simulink model "model_cnn"  (R2020a)
settings: Solver=VariableStepAuto  StartTime=0.0  StopTime=1e6/fs  RelTol=1e-3
PreLoadFcn:
  | setup_imports;
  | %dense2_numerictype = fixdt(1,18,10);
  | %conv1_numerictype = fixdt(1,18,21);
InitFcn:
  | % Intermediate signal dimensions
  | input_dim = [1, 2, 128];
  | layer1_dim = hInterConvLayerDims([1,3,1,64],input_dim,1); % dims : [C,H,W]
  | layer2_dim = hInterConvLayerDims([2,3,64,16],layer1_dim,1);% dims : [C,H,W]
  | layer3_dim = [1,128];
  | 
  | % Conv Layer 1 dimensions
  | conv1_dims = struct(...
  |     'input_dim',    input_dim,...       input_dim = C,H,W
  |     'filter_dim',   [1, 3, 1, 64],...  filter_dim = K,J,C,N
  |     'stride',       1,...
  |     'row_output',   3,...
  |     'output_dim',   layer1_dim);
  | 
  | % Conv Layer 2 dimensions
  | conv2_dims = struct(...
  |     'input_dim',    layer1_dim,...      input = C,H.W
  |     'filter_dim',   [2, 3, 64, 16],...  filter_dim = K,J,C,N
  |     'stride',       1,...
  |     'row_output',   2*3*64,...
  |     'output_dim',   layer2_dim);
  | 
  | % Dense Layer 1 dimensions
  | dense1_dims = struct(...
  |     'input_dim',    layer2_dim,...      input = C,H,W
  |     'weight_dim',   [1984, 128],...     weight_dim = H,W
  |     'output_dim',   layer3_dim);
  | 
  | % Load saved weights and input
  | setup_imports;
  | 
  | fs = 128e6;
  | fs_axi = 100e6;
  | R = 32;
values from neighbouring files (symbols this model uses):
  datatypeInput = X_test.numerictype    [setup_imports.m]
  gemm_wconv1 = fi(hInterleaveFilters(Wconv1),1,16)    [setup_imports.m]
  gemm_wconv2 = fi(hInterleaveFilters(Wconv2),1,16)    [setup_imports.m]
  wdense1 = fi(Wdense1,1,16)    [setup_imports.m]
  wdense2 = fi(Wdense2,1,16)    [setup_imports.m]
undefined symbols (not defined in the file or in its folder): ltehdlRAMinitPO2
libraries: hdlsllib x1022, dspsigops x3, dspsrcs4 x2
(part 22 of 23)

== system model_cnn/HDL CNN Model/Conv Layer 2/Filter Matrix Multiplier1/ParallelMACs 9/MAC10 ==
  countWeights : Inport
  samplesIn : Inport  Port=2
  validIn : Inport  Port=3
  Data Type Conversion : DataTypeConversion  OutDataTypeStr=datatypeLayer2
  Multiply-Accumulate : hdlsllib/HDL Operations/Multiply-Accumulate  opMode=Streaming - using Number of Samples  initValueSetting=Dialog  initValue=0  initValueSetting2=Dialog  initValue2=0  initValueSetting3=Dialog  initValue3=0  num_samples=24  RndMeth2=Floor  RndMeth3=Floor  OutDataTypeStr=gemm_wconv2.numerictype  datatype2=Inherit: Inherit via back propagation  datatype3=accumoutdatatype2  validOut=on  endInandOut=on  startOut=on  countOut=on  dim=-1  DoSatur=off  parallel=off
      settings: SourceProductBaseCode=SL
  Terminator : Terminator
  Terminator1 : Terminator
  Terminator2 : Terminator
  dataOut : Outport
  wires:
  countWeights/1 -> Multiply-Accumulate/2
  ? -> Terminator2/1
  samplesIn/1 -> Multiply-Accumulate/1
  Multiply-Accumulate/1 -> Data Type Conversion/1
  ? -> Terminator/1
  ? -> Terminator1/1
  validIn/1 -> ?
  Data Type Conversion/1 -> dataOut/1

== system model_cnn/HDL CNN Model/Conv Layer 2/Filter Matrix Multiplier1/ParallelMACs 9/MAC11 ==
  countWeights : Inport
  samplesIn : Inport  Port=2
  validIn : Inport  Port=3
  Data Type Conversion : DataTypeConversion  OutDataTypeStr=datatypeLayer2
  Multiply-Accumulate : hdlsllib/HDL Operations/Multiply-Accumulate  opMode=Streaming - using Number of Samples  initValueSetting=Dialog  initValue=0  initValueSetting2=Dialog  initValue2=0  initValueSetting3=Dialog  initValue3=0  num_samples=24  RndMeth2=Floor  RndMeth3=Floor  OutDataTypeStr=gemm_wconv2.numerictype  datatype2=Inherit: Inherit via back propagation  datatype3=accumoutdatatype2  validOut=on  endInandOut=on  startOut=on  countOut=on  dim=-1  DoSatur=off  parallel=off
      settings: SourceProductBaseCode=SL
  Terminator : Terminator
  Terminator1 : Terminator
  Terminator2 : Terminator
  dataOut : Outport
  wires:
  countWeights/1 -> Multiply-Accumulate/2
  ? -> Terminator2/1
  samplesIn/1 -> Multiply-Accumulate/1
  Multiply-Accumulate/1 -> Data Type Conversion/1
  ? -> Terminator/1
  ? -> Terminator1/1
  validIn/1 -> ?
  Data Type Conversion/1 -> dataOut/1

== system model_cnn/HDL CNN Model/Conv Layer 2/Filter Matrix Multiplier1/ParallelMACs 9/MAC12 ==
  countWeights : Inport
  samplesIn : Inport  Port=2
  validIn : Inport  Port=3
  Data Type Conversion : DataTypeConversion  OutDataTypeStr=datatypeLayer2
  Multiply-Accumulate : hdlsllib/HDL Operations/Multiply-Accumulate  opMode=Streaming - using Number of Samples  initValueSetting=Dialog  initValue=0  initValueSetting2=Dialog  initValue2=0  initValueSetting3=Dialog  initValue3=0  num_samples=24  RndMeth2=Floor  RndMeth3=Floor  OutDataTypeStr=gemm_wconv2.numerictype  datatype2=Inherit: Inherit via back propagation  datatype3=accumoutdatatype2  validOut=on  endInandOut=on  startOut=on  countOut=on  dim=-1  DoSatur=off  parallel=off
      settings: SourceProductBaseCode=SL
  Terminator : Terminator
  Terminator1 : Terminator
  Terminator2 : Terminator
  dataOut : Outport
  wires:
  countWeights/1 -> Multiply-Accumulate/2
  ? -> Terminator2/1
  samplesIn/1 -> Multiply-Accumulate/1
  Multiply-Accumulate/1 -> Data Type Conversion/1
  ? -> Terminator/1
  ? -> Terminator1/1
  validIn/1 -> ?
  Data Type Conversion/1 -> dataOut/1

== system model_cnn/HDL CNN Model/Conv Layer 2/Filter Matrix Multiplier1/ParallelMACs 9/MAC13 ==
  countWeights : Inport
  samplesIn : Inport  Port=2
  validIn : Inport  Port=3
  Data Type Conversion : DataTypeConversion  OutDataTypeStr=datatypeLayer2
  Multiply-Accumulate : hdlsllib/HDL Operations/Multiply-Accumulate  opMode=Streaming - using Number of Samples  initValueSetting=Dialog  initValue=0  initValueSetting2=Dialog  initValue2=0  initValueSetting3=Dialog  initValue3=0  num_samples=24  RndMeth2=Floor  RndMeth3=Floor  OutDataTypeStr=gemm_wconv2.numerictype  datatype2=Inherit: Inherit via back propagation  datatype3=accumoutdatatype2  validOut=on  endInandOut=on  startOut=on  countOut=on  dim=-1  DoSatur=off  parallel=off
      settings: SourceProductBaseCode=SL
  Terminator : Terminator
  Terminator1 : Terminator
  Terminator2 : Terminator
  dataOut : Outport
  wires:
  countWeights/1 -> Multiply-Accumulate/2
  ? -> Terminator2/1
  samplesIn/1 -> Multiply-Accumulate/1
  Multiply-Accumulate/1 -> Data Type Conversion/1
  ? -> Terminator/1
  ? -> Terminator1/1
  validIn/1 -> ?
  Data Type Conversion/1 -> dataOut/1

== system model_cnn/HDL CNN Model/Conv Layer 2/Filter Matrix Multiplier1/ParallelMACs 9/MAC14 ==
  countWeights : Inport
  samplesIn : Inport  Port=2
  validIn : Inport  Port=3
  Data Type Conversion : DataTypeConversion  OutDataTypeStr=datatypeLayer2
  Multiply-Accumulate : hdlsllib/HDL Operations/Multiply-Accumulate  opMode=Streaming - using Number of Samples  initValueSetting=Dialog  initValue=0  initValueSetting2=Dialog  initValue2=0  initValueSetting3=Dialog  initValue3=0  num_samples=24  RndMeth2=Floor  RndMeth3=Floor  OutDataTypeStr=gemm_wconv2.numerictype  datatype2=Inherit: Inherit via back propagation  datatype3=accumoutdatatype2  validOut=on  endInandOut=on  startOut=on  countOut=on  dim=-1  DoSatur=off  parallel=off
      settings: SourceProductBaseCode=SL
  Terminator : Terminator
  Terminator1 : Terminator
  Terminator2 : Terminator
  dataOut : Outport
  wires:
  countWeights/1 -> Multiply-Accumulate/2
  ? -> Terminator2/1
  samplesIn/1 -> Multiply-Accumulate/1
  Multiply-Accumulate/1 -> Data Type Conversion/1
  ? -> Terminator/1
  ? -> Terminator1/1
  validIn/1 -> ?
  Data Type Conversion/1 -> dataOut/1

== system model_cnn/HDL CNN Model/Conv Layer 2/Filter Matrix Multiplier1/ParallelMACs 9/MAC15 ==
  countWeights : Inport
  samplesIn : Inport  Port=2
  validIn : Inport  Port=3
  Data Type Conversion : DataTypeConversion  OutDataTypeStr=datatypeLayer2
  Multiply-Accumulate : hdlsllib/HDL Operations/Multiply-Accumulate  opMode=Streaming - using Number of Samples  initValueSetting=Dialog  initValue=0  initValueSetting2=Dialog  initValue2=0  initValueSetting3=Dialog  initValue3=0  num_samples=24  RndMeth2=Floor  RndMeth3=Floor  OutDataTypeStr=gemm_wconv2.numerictype  datatype2=Inherit: Inherit via back propagation  datatype3=accumoutdatatype2  validOut=on  endInandOut=on  startOut=on  countOut=on  dim=-1  DoSatur=off  parallel=off
      settings: SourceProductBaseCode=SL
  Terminator : Terminator
  Terminator1 : Terminator
  Terminator2 : Terminator
  dataOut : Outport
  wires:
  countWeights/1 -> Multiply-Accumulate/2
  ? -> Terminator2/1
  samplesIn/1 -> Multiply-Accumulate/1
  Multiply-Accumulate/1 -> Data Type Conversion/1
  ? -> Terminator/1
  ? -> Terminator1/1
  validIn/1 -> ?
  Data Type Conversion/1 -> dataOut/1

== system model_cnn/HDL CNN Model/Conv Layer 2/Filter Matrix Multiplier1/ParallelMACs 9/MAC2 ==
  countWeights : Inport
  samplesIn : Inport  Port=2
  validIn : Inport  Port=3
  Data Type Conversion : DataTypeConversion  OutDataTypeStr=datatypeLayer2
  Multiply-Accumulate : hdlsllib/HDL Operations/Multiply-Accumulate  opMode=Streaming - using Number of Samples  initValueSetting=Dialog  initValue=0  initValueSetting2=Dialog  initValue2=0  initValueSetting3=Dialog  initValue3=0  num_samples=24  RndMeth2=Floor  RndMeth3=Floor  OutDataTypeStr=gemm_wconv2.numerictype  datatype2=Inherit: Inherit via back propagation  datatype3=accumoutdatatype2  validOut=on  endInandOut=on  startOut=on  countOut=on  dim=-1  DoSatur=off  parallel=off
      settings: SourceProductBaseCode=SL
  Terminator : Terminator
  Terminator1 : Terminator
  Terminator2 : Terminator
  dataOut : Outport
  wires:
  countWeights/1 -> Multiply-Accumulate/2
  ? -> Terminator2/1
  samplesIn/1 -> Multiply-Accumulate/1
  Multiply-Accumulate/1 -> Data Type Conversion/1
  ? -> Terminator/1
  ? -> Terminator1/1
  validIn/1 -> ?
  Data Type Conversion/1 -> dataOut/1

== system model_cnn/HDL CNN Model/Conv Layer 2/Filter Matrix Multiplier1/ParallelMACs 9/MAC3 ==
  countWeights : Inport
  samplesIn : Inport  Port=2
  validIn : Inport  Port=3
  Data Type Conversion : DataTypeConversion  OutDataTypeStr=datatypeLayer2
  Multiply-Accumulate : hdlsllib/HDL Operations/Multiply-Accumulate  opMode=Streaming - using Number of Samples  initValueSetting=Dialog  initValue=0  initValueSetting2=Dialog  initValue2=0  initValueSetting3=Dialog  initValue3=0  num_samples=24  RndMeth2=Floor  RndMeth3=Floor  OutDataTypeStr=gemm_wconv2.numerictype  datatype2=Inherit: Inherit via back propagation  datatype3=accumoutdatatype2  validOut=on  endInandOut=on  startOut=on  countOut=on  dim=-1  DoSatur=off  parallel=off
      settings: SourceProductBaseCode=SL
  Terminator : Terminator
  Terminator1 : Terminator
  Terminator2 : Terminator
  dataOut : Outport
  wires:
  countWeights/1 -> Multiply-Accumulate/2
  ? -> Terminator2/1
  samplesIn/1 -> Multiply-Accumulate/1
  Multiply-Accumulate/1 -> Data Type Conversion/1
  ? -> Terminator/1
  ? -> Terminator1/1
  validIn/1 -> ?
  Data Type Conversion/1 -> dataOut/1

== system model_cnn/HDL CNN Model/Conv Layer 2/Filter Matrix Multiplier1/ParallelMACs 9/MAC4 ==
  countWeights : Inport
  samplesIn : Inport  Port=2
  validIn : Inport  Port=3
  Data Type Conversion : DataTypeConversion  OutDataTypeStr=datatypeLayer2
  Multiply-Accumulate : hdlsllib/HDL Operations/Multiply-Accumulate  opMode=Streaming - using Number of Samples  initValueSetting=Dialog  initValue=0  initValueSetting2=Dialog  initValue2=0  initValueSetting3=Dialog  initValue3=0  num_samples=24  RndMeth2=Floor  RndMeth3=Floor  OutDataTypeStr=gemm_wconv2.numerictype  datatype2=Inherit: Inherit via back propagation  datatype3=accumoutdatatype2  validOut=on  endInandOut=on  startOut=on  countOut=on  dim=-1  DoSatur=off  parallel=off
      settings: SourceProductBaseCode=SL
  Terminator : Terminator
  Terminator1 : Terminator
  Terminator2 : Terminator
  dataOut : Outport
  wires:
  countWeights/1 -> Multiply-Accumulate/2
  ? -> Terminator2/1
  samplesIn/1 -> Multiply-Accumulate/1
  Multiply-Accumulate/1 -> Data Type Conversion/1
  ? -> Terminator/1
  ? -> Terminator1/1
  validIn/1 -> ?
  Data Type Conversion/1 -> dataOut/1

== system model_cnn/HDL CNN Model/Conv Layer 2/Filter Matrix Multiplier1/ParallelMACs 9/MAC5 ==
  countWeights : Inport
  samplesIn : Inport  Port=2
  validIn : Inport  Port=3
  Data Type Conversion : DataTypeConversion  OutDataTypeStr=datatypeLayer2
  Multiply-Accumulate : hdlsllib/HDL Operations/Multiply-Accumulate  opMode=Streaming - using Number of Samples  initValueSetting=Dialog  initValue=0  initValueSetting2=Dialog  initValue2=0  initValueSetting3=Dialog  initValue3=0  num_samples=24  RndMeth2=Floor  RndMeth3=Floor  OutDataTypeStr=gemm_wconv2.numerictype  datatype2=Inherit: Inherit via back propagation  datatype3=accumoutdatatype2  validOut=on  endInandOut=on  startOut=on  countOut=on  dim=-1  DoSatur=off  parallel=off
      settings: SourceProductBaseCode=SL
  Terminator : Terminator
  Terminator1 : Terminator
  Terminator2 : Terminator
  dataOut : Outport
  wires:
  countWeights/1 -> Multiply-Accumulate/2
  ? -> Terminator2/1
  samplesIn/1 -> Multiply-Accumulate/1
  Multiply-Accumulate/1 -> Data Type Conversion/1
  ? -> Terminator/1
  ? -> Terminator1/1
  validIn/1 -> ?
  Data Type Conversion/1 -> dataOut/1

== system model_cnn/HDL CNN Model/Conv Layer 2/Filter Matrix Multiplier1/ParallelMACs 9/MAC6 ==
  countWeights : Inport
  samplesIn : Inport  Port=2
  validIn : Inport  Port=3
  Data Type Conversion : DataTypeConversion  OutDataTypeStr=datatypeLayer2
  Multiply-Accumulate : hdlsllib/HDL Operations/Multiply-Accumulate  opMode=Streaming - using Number of Samples  initValueSetting=Dialog  initValue=0  initValueSetting2=Dialog  initValue2=0  initValueSetting3=Dialog  initValue3=0  num_samples=24  RndMeth2=Floor  RndMeth3=Floor  OutDataTypeStr=gemm_wconv2.numerictype  datatype2=Inherit: Inherit via back propagation  datatype3=accumoutdatatype2  validOut=on  endInandOut=on  startOut=on  countOut=on  dim=-1  DoSatur=off  parallel=off
      settings: SourceProductBaseCode=SL
  Terminator : Terminator
  Terminator1 : Terminator
  Terminator2 : Terminator
  dataOut : Outport
  wires:
  countWeights/1 -> Multiply-Accumulate/2
  ? -> Terminator2/1
  samplesIn/1 -> Multiply-Accumulate/1
  Multiply-Accumulate/1 -> Data Type Conversion/1
  ? -> Terminator/1
  ? -> Terminator1/1
  validIn/1 -> ?
  Data Type Conversion/1 -> dataOut/1

== system model_cnn/HDL CNN Model/Conv Layer 2/Filter Matrix Multiplier1/ParallelMACs 9/MAC7 ==
  countWeights : Inport
  samplesIn : Inport  Port=2
  validIn : Inport  Port=3
  Data Type Conversion : DataTypeConversion  OutDataTypeStr=datatypeLayer2
  Multiply-Accumulate : hdlsllib/HDL Operations/Multiply-Accumulate  opMode=Streaming - using Number of Samples  initValueSetting=Dialog  initValue=0  initValueSetting2=Dialog  initValue2=0  initValueSetting3=Dialog  initValue3=0  num_samples=24  RndMeth2=Floor  RndMeth3=Floor  OutDataTypeStr=gemm_wconv2.numerictype  datatype2=Inherit: Inherit via back propagation  datatype3=accumoutdatatype2  validOut=on  endInandOut=on  startOut=on  countOut=on  dim=-1  DoSatur=off  parallel=off
      settings: SourceProductBaseCode=SL
  Terminator : Terminator
  Terminator1 : Terminator
  Terminator2 : Terminator
  dataOut : Outport
  wires:
  countWeights/1 -> Multiply-Accumulate/2
  ? -> Terminator2/1
  samplesIn/1 -> Multiply-Accumulate/1
  Multiply-Accumulate/1 -> Data Type Conversion/1
  ? -> Terminator/1
  ? -> Terminator1/1
  validIn/1 -> ?
  Data Type Conversion/1 -> dataOut/1

== system model_cnn/HDL CNN Model/Conv Layer 2/Filter Matrix Multiplier1/ParallelMACs 9/MAC8 ==
  countWeights : Inport
  samplesIn : Inport  Port=2
  validIn : Inport  Port=3
  Data Type Conversion : DataTypeConversion  OutDataTypeStr=datatypeLayer2
  Multiply-Accumulate : hdlsllib/HDL Operations/Multiply-Accumulate  opMode=Streaming - using Number of Samples  initValueSetting=Dialog  initValue=0  initValueSetting2=Dialog  initValue2=0  initValueSetting3=Dialog  initValue3=0  num_samples=24  RndMeth2=Floor  RndMeth3=Floor  OutDataTypeStr=gemm_wconv2.numerictype  datatype2=Inherit: Inherit via back propagation  datatype3=accumoutdatatype2  validOut=on  endInandOut=on  startOut=on  countOut=on  dim=-1  DoSatur=off  parallel=off
      settings: SourceProductBaseCode=SL
  Terminator : Terminator
  Terminator1 : Terminator
  Terminator2 : Terminator
  dataOut : Outport
  wires:
  countWeights/1 -> Multiply-Accumulate/2
  ? -> Terminator2/1
  samplesIn/1 -> Multiply-Accumulate/1
  Multiply-Accumulate/1 -> Data Type Conversion/1
  ? -> Terminator/1
  ? -> Terminator1/1
  validIn/1 -> ?
  Data Type Conversion/1 -> dataOut/1

== system model_cnn/HDL CNN Model/Conv Layer 2/Filter Matrix Multiplier1/ParallelMACs 9/MAC9 ==
  countWeights : Inport
  samplesIn : Inport  Port=2
  validIn : Inport  Port=3
  Data Type Conversion : DataTypeConversion  OutDataTypeStr=datatypeLayer2
  Multiply-Accumulate : hdlsllib/HDL Operations/Multiply-Accumulate  opMode=Streaming - using Number of Samples  initValueSetting=Dialog  initValue=0  initValueSetting2=Dialog  initValue2=0  initValueSetting3=Dialog  initValue3=0  num_samples=24  RndMeth2=Floor  RndMeth3=Floor  OutDataTypeStr=gemm_wconv2.numerictype  datatype2=Inherit: Inherit via back propagation  datatype3=accumoutdatatype2  validOut=on  endInandOut=on  startOut=on  countOut=on  dim=-1  DoSatur=off  parallel=off
      settings: SourceProductBaseCode=SL
  Terminator : Terminator
  Terminator1 : Terminator
  Terminator2 : Terminator
  dataOut : Outport
  wires:
  countWeights/1 -> Multiply-Accumulate/2
  ? -> Terminator2/1
  samplesIn/1 -> Multiply-Accumulate/1
  Multiply-Accumulate/1 -> Data Type Conversion/1
  ? -> Terminator/1
  ? -> Terminator1/1
  validIn/1 -> ?
  Data Type Conversion/1 -> dataOut/1

== system model_cnn/HDL CNN Model/Conv Layer 2/Filter Matrix Multiplier1/ParallelMACs 9/Weight Storage 0 ==
  count_Weights : Inport
  Constant : Constant  Value=0  OutDataTypeStr=gemm_wconv2.numerictype  SampleTime=-1
  Constant1 : Constant  Value=false  SampleTime=-1
  Single Port RAM System : hdlsllib/HDL RAMs/Single Port RAM System  RAMType=Single port  WriteOutputValue=New data  RAMInitialValue=[gemm_wconv2(dim,(dim2:16:16*24)),zeros(1,8)]  SimulateUsing=Code generation
      settings: SourceProductBaseCode=SL
  weightsOut : Outport
  wires:
  count_Weights/1 -> Single Port RAM System/2
  Constant1/1 -> Single Port RAM System/3
  Constant/1 -> Single Port RAM System/1
  Single Port RAM System/1 -> weightsOut/1

== system model_cnn/HDL CNN Model/Conv Layer 2/Filter Matrix Multiplier1/ParallelMACs 9/Weight Storage1 ==
  count_Weights : Inport
  Constant : Constant  Value=0  OutDataTypeStr=gemm_wconv2.numerictype  SampleTime=-1
  Constant1 : Constant  Value=false  SampleTime=-1
  Single Port RAM System : hdlsllib/HDL RAMs/Single Port RAM System  RAMType=Single port  WriteOutputValue=New data  RAMInitialValue=[gemm_wconv2(dim,(dim2:16:16*24)),zeros(1,8)]  SimulateUsing=Code generation
      settings: SourceProductBaseCode=SL
  weightsOut : Outport
  wires:
  Single Port RAM System/1 -> weightsOut/1
  Constant/1 -> Single Port RAM System/1
  Constant1/1 -> Single Port RAM System/3
  count_Weights/1 -> Single Port RAM System/2

== system model_cnn/HDL CNN Model/Conv Layer 2/Filter Matrix Multiplier1/ParallelMACs 9/Weight Storage10 ==
  count_Weights : Inport
  Constant : Constant  Value=0  OutDataTypeStr=gemm_wconv2.numerictype  SampleTime=-1
  Constant1 : Constant  Value=false  SampleTime=-1
  Single Port RAM System : hdlsllib/HDL RAMs/Single Port RAM System  RAMType=Single port  WriteOutputValue=New data  RAMInitialValue=[gemm_wconv2(dim,(dim2:16:16*24)),zeros(1,8)]  SimulateUsing=Code generation
      settings: SourceProductBaseCode=SL
  weightsOut : Outport
  wires:
  Single Port RAM System/1 -> weightsOut/1
  Constant/1 -> Single Port RAM System/1
  Constant1/1 -> Single Port RAM System/3
  count_Weights/1 -> Single Port RAM System/2

== system model_cnn/HDL CNN Model/Conv Layer 2/Filter Matrix Multiplier1/ParallelMACs 9/Weight Storage11 ==
  count_Weights : Inport
  Constant : Constant  Value=0  OutDataTypeStr=gemm_wconv2.numerictype  SampleTime=-1
  Constant1 : Constant  Value=false  SampleTime=-1
  Single Port RAM System : hdlsllib/HDL RAMs/Single Port RAM System  RAMType=Single port  WriteOutputValue=New data  RAMInitialValue=[gemm_wconv2(dim,(dim2:16:16*24)),zeros(1,8)]  SimulateUsing=Code generation
      settings: SourceProductBaseCode=SL
  weightsOut : Outport
  wires:
  Single Port RAM System/1 -> weightsOut/1
  Constant/1 -> Single Port RAM System/1
  Constant1/1 -> Single Port RAM System/3
  count_Weights/1 -> Single Port RAM System/2

== system model_cnn/HDL CNN Model/Conv Layer 2/Filter Matrix Multiplier1/ParallelMACs 9/Weight Storage12 ==
  count_Weights : Inport
  Constant : Constant  Value=0  OutDataTypeStr=gemm_wconv2.numerictype  SampleTime=-1
  Constant1 : Constant  Value=false  SampleTime=-1
  Single Port RAM System : hdlsllib/HDL RAMs/Single Port RAM System  RAMType=Single port  WriteOutputValue=New data  RAMInitialValue=[gemm_wconv2(dim,(dim2:16:16*24)),zeros(1,8)]  SimulateUsing=Code generation
      settings: SourceProductBaseCode=SL
  weightsOut : Outport
  wires:
  Single Port RAM System/1 -> weightsOut/1
  Constant/1 -> Single Port RAM System/1
  Constant1/1 -> Single Port RAM System/3
  count_Weights/1 -> Single Port RAM System/2

== system model_cnn/HDL CNN Model/Conv Layer 2/Filter Matrix Multiplier1/ParallelMACs 9/Weight Storage13 ==
  count_Weights : Inport
  Constant : Constant  Value=0  OutDataTypeStr=gemm_wconv2.numerictype  SampleTime=-1
  Constant1 : Constant  Value=false  SampleTime=-1
  Single Port RAM System : hdlsllib/HDL RAMs/Single Port RAM System  RAMType=Single port  WriteOutputValue=New data  RAMInitialValue=[gemm_wconv2(dim,(dim2:16:16*24)),zeros(1,8)]  SimulateUsing=Code generation
      settings: SourceProductBaseCode=SL
  weightsOut : Outport
  wires:
  Single Port RAM System/1 -> weightsOut/1
  Constant/1 -> Single Port RAM System/1
  Constant1/1 -> Single Port RAM System/3
  count_Weights/1 -> Single Port RAM System/2

== system model_cnn/HDL CNN Model/Conv Layer 2/Filter Matrix Multiplier1/ParallelMACs 9/Weight Storage14 ==
  count_Weights : Inport
  Constant : Constant  Value=0  OutDataTypeStr=gemm_wconv2.numerictype  SampleTime=-1
  Constant1 : Constant  Value=false  SampleTime=-1
  Single Port RAM System : hdlsllib/HDL RAMs/Single Port RAM System  RAMType=Single port  WriteOutputValue=New data  RAMInitialValue=[gemm_wconv2(dim,(dim2:16:16*24)),zeros(1,8)]  SimulateUsing=Code generation
      settings: SourceProductBaseCode=SL
  weightsOut : Outport
  wires:
  Single Port RAM System/1 -> weightsOut/1
  Constant/1 -> Single Port RAM System/1
  Constant1/1 -> Single Port RAM System/3
  count_Weights/1 -> Single Port RAM System/2

== system model_cnn/HDL CNN Model/Conv Layer 2/Filter Matrix Multiplier1/ParallelMACs 9/Weight Storage15 ==
  count_Weights : Inport
  Constant : Constant  Value=0  OutDataTypeStr=gemm_wconv2.numerictype  SampleTime=-1
  Constant1 : Constant  Value=false  SampleTime=-1
  Single Port RAM System : hdlsllib/HDL RAMs/Single Port RAM System  RAMType=Single port  WriteOutputValue=New data  RAMInitialValue=[gemm_wconv2(dim,(dim2:16:16*24)),zeros(1,8)]  SimulateUsing=Code generation
      settings: SourceProductBaseCode=SL
  weightsOut : Outport
  wires:
  Single Port RAM System/1 -> weightsOut/1
  Constant/1 -> Single Port RAM System/1
  Constant1/1 -> Single Port RAM System/3
  count_Weights/1 -> Single Port RAM System/2

== system model_cnn/HDL CNN Model/Conv Layer 2/Filter Matrix Multiplier1/ParallelMACs 9/Weight Storage2 ==
  count_Weights : Inport
  Constant : Constant  Value=0  OutDataTypeStr=gemm_wconv2.numerictype  SampleTime=-1
  Constant1 : Constant  Value=false  SampleTime=-1
  Single Port RAM System : hdlsllib/HDL RAMs/Single Port RAM System  RAMType=Single port  WriteOutputValue=New data  RAMInitialValue=[gemm_wconv2(dim,(dim2:16:16*24)),zeros(1,8)]  SimulateUsing=Code generation
      settings: SourceProductBaseCode=SL
  weightsOut : Outport
  wires:
  Single Port RAM System/1 -> weightsOut/1
  Constant/1 -> Single Port RAM System/1
  Constant1/1 -> Single Port RAM System/3
  count_Weights/1 -> Single Port RAM System/2

== system model_cnn/HDL CNN Model/Conv Layer 2/Filter Matrix Multiplier1/ParallelMACs 9/Weight Storage3 ==
  count_Weights : Inport
  Constant : Constant  Value=0  OutDataTypeStr=gemm_wconv2.numerictype  SampleTime=-1
  Constant1 : Constant  Value=false  SampleTime=-1
  Single Port RAM System : hdlsllib/HDL RAMs/Single Port RAM System  RAMType=Single port  WriteOutputValue=New data  RAMInitialValue=[gemm_wconv2(dim,(dim2:16:16*24)),zeros(1,8)]  SimulateUsing=Code generation
      settings: SourceProductBaseCode=SL
  weightsOut : Outport
  wires:
  Single Port RAM System/1 -> weightsOut/1
  Constant/1 -> Single Port RAM System/1
  Constant1/1 -> Single Port RAM System/3
  count_Weights/1 -> Single Port RAM System/2

== system model_cnn/HDL CNN Model/Conv Layer 2/Filter Matrix Multiplier1/ParallelMACs 9/Weight Storage4 ==
  count_Weights : Inport
  Constant : Constant  Value=0  OutDataTypeStr=gemm_wconv2.numerictype  SampleTime=-1
  Constant1 : Constant  Value=false  SampleTime=-1
  Single Port RAM System : hdlsllib/HDL RAMs/Single Port RAM System  RAMType=Single port  WriteOutputValue=New data  RAMInitialValue=[gemm_wconv2(dim,(dim2:16:16*24)),zeros(1,8)]  SimulateUsing=Code generation
      settings: SourceProductBaseCode=SL
  weightsOut : Outport
  wires:
  Single Port RAM System/1 -> weightsOut/1
  Constant/1 -> Single Port RAM System/1
  Constant1/1 -> Single Port RAM System/3
  count_Weights/1 -> Single Port RAM System/2

== system model_cnn/HDL CNN Model/Conv Layer 2/Filter Matrix Multiplier1/ParallelMACs 9/Weight Storage5 ==
  count_Weights : Inport
  Constant : Constant  Value=0  OutDataTypeStr=gemm_wconv2.numerictype  SampleTime=-1
  Constant1 : Constant  Value=false  SampleTime=-1
  Single Port RAM System : hdlsllib/HDL RAMs/Single Port RAM System  RAMType=Single port  WriteOutputValue=New data  RAMInitialValue=[gemm_wconv2(dim,(dim2:16:16*24)),zeros(1,8)]  SimulateUsing=Code generation
      settings: SourceProductBaseCode=SL
  weightsOut : Outport
  wires:
  Single Port RAM System/1 -> weightsOut/1
  Constant/1 -> Single Port RAM System/1
  Constant1/1 -> Single Port RAM System/3
  count_Weights/1 -> Single Port RAM System/2

== system model_cnn/HDL CNN Model/Conv Layer 2/Filter Matrix Multiplier1/ParallelMACs 9/Weight Storage6 ==
  count_Weights : Inport
  Constant : Constant  Value=0  OutDataTypeStr=gemm_wconv2.numerictype  SampleTime=-1
  Constant1 : Constant  Value=false  SampleTime=-1
  Single Port RAM System : hdlsllib/HDL RAMs/Single Port RAM System  RAMType=Single port  WriteOutputValue=New data  RAMInitialValue=[gemm_wconv2(dim,(dim2:16:16*24)),zeros(1,8)]  SimulateUsing=Code generation
      settings: SourceProductBaseCode=SL
  weightsOut : Outport
  wires:
  Single Port RAM System/1 -> weightsOut/1
  Constant/1 -> Single Port RAM System/1
  Constant1/1 -> Single Port RAM System/3
  count_Weights/1 -> Single Port RAM System/2

== system model_cnn/HDL CNN Model/Conv Layer 2/Filter Matrix Multiplier1/ParallelMACs 9/Weight Storage7 ==
  count_Weights : Inport
  Constant : Constant  Value=0  OutDataTypeStr=gemm_wconv2.numerictype  SampleTime=-1
  Constant1 : Constant  Value=false  SampleTime=-1
  Single Port RAM System : hdlsllib/HDL RAMs/Single Port RAM System  RAMType=Single port  WriteOutputValue=New data  RAMInitialValue=[gemm_wconv2(dim,(dim2:16:16*24)),zeros(1,8)]  SimulateUsing=Code generation
      settings: SourceProductBaseCode=SL
  weightsOut : Outport
  wires:
  Single Port RAM System/1 -> weightsOut/1
  Constant/1 -> Single Port RAM System/1
  Constant1/1 -> Single Port RAM System/3
  count_Weights/1 -> Single Port RAM System/2

== system model_cnn/HDL CNN Model/Conv Layer 2/Filter Matrix Multiplier1/ParallelMACs 9/Weight Storage8 ==
  count_Weights : Inport
  Constant : Constant  Value=0  OutDataTypeStr=gemm_wconv2.numerictype  SampleTime=-1
  Constant1 : Constant  Value=false  SampleTime=-1
  Single Port RAM System : hdlsllib/HDL RAMs/Single Port RAM System  RAMType=Single port  WriteOutputValue=New data  RAMInitialValue=[gemm_wconv2(dim,(dim2:16:16*24)),zeros(1,8)]  SimulateUsing=Code generation
      settings: SourceProductBaseCode=SL
  weightsOut : Outport
  wires:
  Single Port RAM System/1 -> weightsOut/1
  Constant/1 -> Single Port RAM System/1
  Constant1/1 -> Single Port RAM System/3
  count_Weights/1 -> Single Port RAM System/2

== system model_cnn/HDL CNN Model/Conv Layer 2/Filter Matrix Multiplier1/ParallelMACs 9/Weight Storage9 ==
  count_Weights : Inport
  Constant : Constant  Value=0  OutDataTypeStr=gemm_wconv2.numerictype  SampleTime=-1
  Constant1 : Constant  Value=false  SampleTime=-1
  Single Port RAM System : hdlsllib/HDL RAMs/Single Port RAM System  RAMType=Single port  WriteOutputValue=New data  RAMInitialValue=[gemm_wconv2(dim,(dim2:16:16*24)),zeros(1,8)]  SimulateUsing=Code generation
      settings: SourceProductBaseCode=SL
  weightsOut : Outport
  wires:
  Single Port RAM System/1 -> weightsOut/1
  Constant/1 -> Single Port RAM System/1
  Constant1/1 -> Single Port RAM System/3
  count_Weights/1 -> Single Port RAM System/2

== matlab function model_cnn/HDL CNN Model/Conv Layer 2/ReLU ==
  data: in input; out output
function out = ReLU(in)
% Perform the ReLU activation function. 

%     relu = max(cast(0,'like',in),in);
%     clip = fi(relu,1,2,1);
%     out  = relu;
    relu = max(fi(0,1,16,14),fi(in,1,16,14));
%     clip = fi(relu,1,2,1);
    out  = relu;
end

== matlab function model_cnn/HDL CNN Model/Conv Layer 2/Vector Slice Selection/Frame Slicer1 ==
  data: frameIn input; slicedFrame output
function slicedFrame = frame_slicer(frameIn)

    slicedFrame = cast(zeros(16,1),'like',frameIn);
    slicedFrame(:) = frameIn(17:32);

end

== matlab function model_cnn/HDL CNN Model/Conv Layer 2/Vector Slice Selection/Frame Slicer2 ==
  data: frameIn input; slicedFrame output
function slicedFrame = frame_slicer(frameIn)
    
    slicedFrame = cast(zeros(16,1),'like',frameIn);
    slicedFrame(:) = frameIn(33:48);

end

== matlab function model_cnn/HDL CNN Model/Conv Layer 2/Vector Slice Selection/Frame Slicer3 ==
  data: frameIn input; slicedFrame output
function slicedFrame = frame_slicer(frameIn)

    slicedFrame = cast(zeros(16,1),'like',frameIn);
    slicedFrame(:) = frameIn(49:64);

end

== matlab function model_cnn/HDL CNN Model/Conv Layer 1/ReLU ==
  data: in input; out output
function out = ReLU(in)
% Perform the ReLU activation function. 

%     relu = max(fi(0,in.numerictype),in);
    relu = max(fi(0,1,16,14),fi(in,1,16,14));
%     clip = fi(relu,1,2,1);
    out  = relu;
    
end
%     clip = fi(relu,1,2,1);https://github.com/axdy/rfsoc_quant_amc

== matlab function model_cnn/HDL CNN Model/Dense Layer 1/ReLU 3 ==
  data: in input; out output
function out = ReLU(in)
% Perform the ReLU activation function. 

%     relu = max(fi(0,in.numerictype),in);
%     relu = max(fi(0,1,16,0),fi(in,1,16,0));
% %     clip = fi(relu,1,2,1);
%     out  = relu;
    relu = max(fi(0,1,16,12),fi(in,1,16,12));
%     clip = fi(relu,1,2,1);
    out  = relu;
    
    
end

== matlab function model_cnn/HDL CNN Model/Conv Layer 2/Buffer and Sliding Window State Machine ==
  data: wr_addr output; wr_en output; rd_addr output; rd_row_idx output; validIn input; ready_nx_layer input; validOut output; ready_prev output; conv2_dims parameter
function [wr_addr, wr_en, rd_addr, rd_row_idx, validOut, ready_prev] = buffer_sliding_window(validIn, ready_nx_layer, conv2_dims)
%#codegen

    persistent reg state sw_reg buffer
    
    % States
    IDLE_STATE = 0;
    WRITE_SAMPLES_STATE = 1;    % Write samples to buffer
    READ_SAMPLES_STATE = 2;
    WAIT_TO_SLIDE_STATE = 3;	% Wait for ready to perform sliding window
    SLIDING_WINDOW_STATE = 4;   % Slide window for next layer input
    
    % Constant Variables
    addr_length = prod(conv2_dims.input_dim);
    input_dim = conv2_dims.input_dim;
    filter_dim = conv2_dims.filter_dim;
    outdim = conv2_dims.output_dim;
    row_output = conv2_dims.row_output;
    input_row = conv2_dims.input_dim(1);
    input_cols = conv2_dims.input_dim(2)*conv2_dims.input_dim(3);
    swu_total_length = conv2_dims.row_output * conv2_dims.output_dim(3);
    
    
    if isempty(state)
        state = fi(0,0,3,0);
        state(:) = WRITE_SAMPLES_STATE;
    end
    
    if isempty(reg)
        reg = struct(...
            'data_count',   fi(0,0,ceil(log2(addr_length)),0,hdlfimath),... Counting to 252*64
            'wr_addr',      fi(0,0,ceil(log2(addr_length)),0,hdlfimath),...
            'rd_addr',      fi(0,0,ceil(log2(addr_length)),0,hdlfimath),...
            'wr_en',        false,...
            'ready_nx_layer', false,...
            'validOut',     false,...
            'flag',         false,...
            'ready_flag',   true,...
            'input_count',  fi(0,0,ceil(log2(input_cols)+1),0,hdlfimath),...
            'buffer_idx',   fi(0,0,ceil(log2(input_row)+1),0,hdlfimath),...
            'count_out_cols', fi(0,0,ceil(log2(input_cols)+1),0,hdlfimath),...
            'repeat_frame', fi(0,0,3,0,hdlfimath),...
            'track_stored', fi(0,0,ceil(log2(input_cols)+1),0,hdlfimath));
    end
    
    if isempty(sw_reg)
        sw_reg = struct(...
            'i',            fi(0,0,ceil(log2(outdim(2)))+1,0,hdlfimath),... I = 1 (output dim y)
            'j',            fi(0,0,ceil(log2(outdim(3)))+1,0,hdlfimath),... J = 124 (output dim x)
            'a',            fi(0,0,ceil(log2(filter_dim(1)))+1,0,hdlfimath),... A = 2
            'b',            fi(0,0,ceil(log2(filter_dim(2)))+1,0,hdlfimath),... B = 3
            'c',            fi(0,0,ceil(log2(filter_dim(3)))+1,0,hdlfimath),... C = 64
            'row_count',    fi(0,0,ceil(log2(row_output))+1,0,hdlfimath),... row out = 64*2*3
            'flag',         true);
    end
    
    if isempty(buffer)
        buffer = fi(zeros(input_row,input_cols),1,16,19);
    end
    
    validOut = false;
    rd_addr = fi(0,0,ceil(log2(input_cols)+1),0,hdlfimath);
    wr_addr = fi(0,0,ceil(log2(input_cols)+1),0,hdlfimath);
    wr_en = false;
    ready_prev = false;
    rd_row_idx = fi(0,0,ceil(log2(input_row)+1),0,hdlfimath);
    
    switch state
        case WRITE_SAMPLES_STATE
            if validIn
                wr_en = true;
                wr_addr(:) = reg.input_count;
                reg.track_stored(:) = reg.track_stored + 1;
                reg.flag = true;
                if reg.input_count == input_cols - 1
                    reg.input_count(:) = 0;
                else
                    reg.input_count(:) = reg.input_count + 1;
                end
            end
            
            if ready_nx_layer && ~reg.ready_nx_layer
                reg.ready_flag = true;
            end
            
            if reg.flag && reg.ready_flag
                if reg.count_out_cols < reg.track_stored
                    % Sliding window operation for GEMM transform for next layer
                    stride_C = fi(input_dim(1),0,ceil(log2(input_dim(1)))+1,0);
                    stride_K_C = fi(input_dim(2)*input_dim(1),0,ceil(log2(input_dim(2)*input_dim(1)))+1,0);
    %                 rd_addr = cast(((sw_reg.i + sw_reg.a) * stride_C) + sw_reg.c + ...
    %                         ((sw_reg.j + sw_reg.b) * stride_K_C),'like',reg.rd_addr);

                    reg.count_out_cols(:) = cast((sw_reg.i + sw_reg.a) + ...
                            ((sw_reg.j + sw_reg.b) * 2),'like',reg.rd_addr);

                    rd_addr(:) = reg.count_out_cols;

                    rd_row_idx(:) = sw_reg.c;

                    validOut = true;
                    
                    if reg.repeat_frame == (4-1)
                        reg.repeat_frame(:) = 0;
                        % loop over kernel y direction
                        if sw_reg.b == (filter_dim(2)-1) % SAME HERE
                            sw_reg.b(:) = 0;

                            % loop over kernel x direction
                            if sw_reg.a == (filter_dim(1)-1) % AND HERE
                                sw_reg.a(:) = 0;

                                % loop over input y direction
                                if sw_reg.i == (outdim(2)-1) % AND HERE
                                    sw_reg.i(:) = 0;

                                    % loop over input x direction
                                    if sw_reg.j == (outdim(3)-1) % AND HERE
                                        sw_reg.j(:) = 0;

                                        ready_prev = true;
                                        reg.flag = false;
                                        reg.ready_flag = false;
                                        reg.track_stored(:) = 0;    % Reset to zero
                                    else
                                        sw_reg.j(:) = sw_reg.j(:) + 1;
                                    end
                                else
                                    sw_reg.i(:) = sw_reg.i(:) + 1;
                                end
                            else
                                sw_reg.a(:) = sw_reg.a + 1;
                            end
                        else
                            sw_reg.b(:) = sw_reg.b + 1;
                        end
                    else
                        reg.repeat_frame(:) = reg.repeat_frame + 1;
                    end
                else
                    validOut = false;
                end
            end
    end
    
    reg.ready_nx_layer = ready_nx_layer;
end

== matlab function model_cnn/HDL CNN Model/Conv Layer 1/Buffer and Sliding Window State Machine ==
  data: validIn input; wr_addr output; wr_en output; enable input; rd_addr output; validOut output; ready_nx_layer input; conv1_dims parameter
function [wr_addr, wr_en, rd_addr, validOut] = bram_controller(validIn,enable,ready_nx_layer,conv1_dims)
%#codegen

    
    persistent reg state sw_reg
    
    % States
    IDLE_STATE = 0;
    WRITE_SAMPLES_STATE = 1;    % Write samples to buffer
    READ_SAMPLES_STATE = 2;
    WAIT_TO_SLIDE_STATE = 3;	% Wait for ready to perform sliding window
    SLIDING_WINDOW_STATE = 4;   % Slide window for next layer input
    
    % Constant Variables
    addr_length = prod(conv1_dims.input_dim);
    input_dim = conv1_dims.input_dim;
    filter_dim = conv1_dims.filter_dim;
    outdim = conv1_dims.output_dim;
    row_output = conv1_dims.row_output;
    
    if isempty(state)
        state = fi(0,0,3,0);
        state(:) = IDLE_STATE;
    end
    
    if isempty(reg)
        reg = struct(...
            'data_count',   fi(0,0,ceil(log2(addr_length)),0,hdlfimath),...
            'wr_addr',      fi(0,0,ceil(log2(addr_length)),0,hdlfimath),...
            'rd_addr',      fi(0,0,ceil(log2(addr_length)),0,hdlfimath),...
            'wr_en',        false,...
            'ready',        false,...
            'ready_nx_layer', true,...
            'validOut',     false,...
            'flag',         false);
    end
    
    if isempty(sw_reg)
        sw_reg = struct(...
            'i',            fi(0,0,ceil(log2(outdim(2))),0,hdlfimath),...   i : outdim_y
            'j',            fi(0,0,ceil(log2(outdim(3))),0,hdlfimath),...   j : outdim_x
            'a',            fi(0,0,ceil(log2(filter_dim(1))),0,hdlfimath),...   a : kernel_y
            'b',            fi(0,0,ceil(log2(filter_dim(2))),0,hdlfimath),...   b : kernel_x
            'row_count',    fi(0,0,ceil(log2(row_output)),0,hdlfimath),...
            'flag',         true);
    end
    
    wr_en = false;
    wr_addr = fi(0,0,ceil(log2(addr_length)),0,hdlfimath);
    validOut = false;
    rd_addr = fi(0,0,ceil(log2(addr_length)),0,hdlfimath);
    
    if ready_nx_layer
        reg.ready_nx_layer = true;
    end
    
    switch state
        case IDLE_STATE
            if enable
                state(:) = WRITE_SAMPLES_STATE;
                if validIn
                    reg.wr_en = true;
                    reg.wr_addr = reg.data_count;
                    reg.data_count(:) = reg.data_count + 1;
                else
                    reg.wr_en = false;                    
                end
                wr_en = reg.wr_en;
            end
            
        case WRITE_SAMPLES_STATE
            if validIn
                if reg.data_count == addr_length-1
                    reg.flag = true;
                    reg.wr_addr = reg.data_count;
                    reg.data_count(:) = reg.data_count + 1;
                    reg.wr_en = true;
                else
                    reg.wr_addr = reg.data_count;
                    reg.data_count(:) = reg.data_count + 1;
                    reg.wr_en = true;                    
                end
                wr_en = reg.wr_en;
                wr_addr = reg.wr_addr;
            end
            
            if reg.flag
                if reg.ready_nx_layer
                    state(:) = SLIDING_WINDOW_STATE;%WAIT_TO_SLIDE_STATE;
                    reg.data_count(:) = 0;
                    reg.flag = false;
                    sw_reg.flag = true;
                    reg.ready_nx_layer = false;
                end
            end
       
        case READ_SAMPLES_STATE
            if reg.data_count == 255
                reg.rd_addr = reg.data_count;
                reg.data_count(:) = reg.data_count + 1;
                reg.wr_en = false;
                reg.validOut = true;
                state(:) = IDLE_STATE;
            else
                reg.flag = false;
                reg.rd_addr = reg.data_count;
                reg.data_count(:) = reg.data_count + 1;
                reg.wr_en = false;
                reg.validOut = true;
            end
            wr_en = reg.wr_en;
            rd_addr = reg.rd_addr;
            validOut = reg.validOut;
       
        case WAIT_TO_SLIDE_STATE
                state(:) = SLIDING_WINDOW_STATE;
                reg.validOut = false;
        
        case SLIDING_WINDOW_STATE
            
            % Sliding window operation for GEMM transform for next layer
            stride_x = fi(input_dim(2),0,ceil(log2(input_dim(2)))+1,0); % not the same stride for kernel. This is for 2D access on 1D array
            % To access a 1D array in memory like a 2D matrix
            rd_addr = cast(((sw_reg.j + sw_reg.b) * stride_x) + ...
                        (sw_reg.i + sw_reg.a),'like',reg.rd_addr);
            
            validOut = false;
             
            if sw_reg.flag
                validOut = true;
                % loop over kernel x direction
                if sw_reg.b == (filter_dim(2)-1) % CHANGE THIS VALUE TO BE PRECALCUALTED
                    sw_reg.b(:) = 0;

                    % loop over kernel y direction
                    if sw_reg.a == (filter_dim(1)-1) % SAME HERE
                        sw_reg.a(:) = 0;

                        % loop over input y direction
                        if sw_reg.i == (outdim(2)-1) % AND HERE
                            sw_reg.i(:) = 0;

                            % loop over input x direction
                            if sw_reg.j == (outdim(3)-1) % AND HERE
                                sw_reg.j(:) = 0;

                                state(:) = WRITE_SAMPLES_STATE;
                                sw_reg.flag = false;
                            else
                                sw_reg.j(:) = sw_reg.j(:) + 1;
                            end
                        else
                            sw_reg.i(:) = sw_reg.i + 1;
                        end
                    else
                        sw_reg.a(:) = sw_reg.a + 1;
                    end
                else
                    sw_reg.b(:) = sw_reg.b + 1;
                end
            end
    end
    
    reg.ready = enable;
end

== matlab function model_cnn/HDL CNN Model/Dense Layer 1/Sample Storage Buffer1 ==
  data: wr_addr output; wr_en output; rd_addr output; rd_row_idx output; validIn input; validOut output; ready_prev output; dense1_dims parameter
function [wr_addr, wr_en, rd_addr, rd_row_idx, validOut, ready_prev] = buffer_sliding_window(validIn,dense1_dims)
%#codegen

    persistent reg state sw_reg
    
    % States
    WRITE_SAMPLES_STATE = 1;    % Write samples to buffer
    
    % Constant Variables
    input_row = dense1_dims.input_dim(1);
    input_cols = dense1_dims.input_dim(2)*dense1_dims.input_dim(3);
    
    
    if isempty(state)
        state = fi(0,0,3,0);
        state(:) = WRITE_SAMPLES_STATE;
    end
    
    if isempty(reg)
        reg = struct(...
            'wr_en',        false,...
            'ready_nx_layer', false,...
            'validOut',     false,...
            'flag',         false,...
            'input_count',  fi(0,0,ceil(log2(input_cols)+1),0,hdlfimath),...
            'buffer_idx',   fi(0,0,ceil(log2(input_row)+1),0,hdlfimath),...
            'count_out_rows', fi(0,0,ceil(log2(input_row)+1),0,hdlfimath),...
            'count_out_cols', fi(0,0,ceil(log2(input_cols)+1),0,hdlfimath),...
            'track_stored', fi(0,0,ceil(log2(input_cols)+1),0,hdlfimath));
    end
    
    if isempty(sw_reg)
        sw_reg = struct(...
            'flag',         true);
    end
    
    validOut = false;
    rd_addr = fi(0,0,ceil(log2(input_cols)+1),0,hdlfimath);
    wr_addr = fi(0,0,ceil(log2(input_cols)+1),0,hdlfimath);
    wr_en = false;
    ready_prev = false;
    rd_row_idx = fi(0,0,ceil(log2(input_row)+1),0,hdlfimath);
    
    switch state
        case WRITE_SAMPLES_STATE
            if validIn
                wr_en = true;
                wr_addr(:) = reg.input_count;
                reg.track_stored(:) = reg.track_stored + 1;     % tracks how many samples have been stored in memory
                reg.flag = true;
                if reg.input_count == input_cols - 1
                    reg.input_count(:) = 0;
                else
                    reg.input_count(:) = reg.input_count + 1;
                end
            end
            
            if reg.flag % and ready_nx_layer
                if reg.count_out_cols < reg.track_stored
                    rd_addr(:) = reg.count_out_cols;

                    rd_row_idx(:) = reg.count_out_rows;

                    validOut = true;

                    if reg.count_out_rows == input_row-1 
                        reg.count_out_rows(:) = 0;
                        if reg.count_out_cols == input_cols-1
                            reg.count_out_cols(:) = 0;
                            reg.track_stored(:) = 0;
                            ready_prev = true;
                            reg.flag = false;
                        else
                            reg.count_out_cols(:) = reg.count_out_cols + 1;
                        end
                    else
                        reg.count_out_rows(:) = reg.count_out_rows + 1;
                    end                    
                end
            else
                validOut = false;
            end
    end
    
end

== matlab function model_cnn/HDL CNN Model/Conv Layer 2/Vector Slice Selection/Frame Slicer ==
  data: frameIn input; slicedFrame output
function slicedFrame = frame_slicer(frameIn)

    slicedFrame = cast(zeros(16,1),'like',frameIn);
    slicedFrame(:) = frameIn(1:16);

end

== matlab function model_cnn/HDL CNN Model/Dense Layer 1/Output Buffer1 ==
  data: vectorIn input; samplesOut output; validIn input; validOut output; done output boolean
function [samplesOut, validOut, done]  = output_buffer(vectorIn, validIn)

    vector_size = 128;
    persistent reg buffer
    
    if isempty(reg)
        reg = struct(...
            'validOut',     false,...
            'flag',         false,...
            'count_out',    fi(0,0,ceil(log2(vector_size))+1,0,hdlfimath));   % for a vector of 16
    end
    
    if isempty(buffer)
%         buffer = fi(zeros(vector_size,1),1,16,15);
        buffer = fi(zeros(vector_size,1),vectorIn.numerictype);
    end

    if validIn
        reg.flag = true;
        buffer(:) = vectorIn;
        reg.count_out(:) = 0;
    end
    
    done = logical(false);
    
    if reg.flag
        samplesOut = buffer(reg.count_out+1);
        reg.count_out(:) = reg.count_out + 1;
        validOut = true;
        if reg.count_out == vector_size
            reg.flag = false;
            done = true;
        end
    else
        reg.count_out(:) = 0;
        reg.flag = false;
        samplesOut = fi(0,vectorIn.numerictype);
        validOut = false;
    end
    
end
